simulink model "non_recursive"  (Simulink 9.1)
settings: Solver=VariableStepDiscrete  StartTime=0.0  StopTime=20.0  RelTol=1e-3  EnableMultiTasking=on
settings Model: Creator=Admin  LastModifiedBy=Asus
settings DataIOCC: LimitDataPoints=on  SignalLoggingSaveFormat=ModelDataLogs
settings OptimizationCC: ExpressionDepthLimit=2147483647  InitFltsAndDblsToZero=on
settings DebuggingCC: SaveWithParameterizedLinksMsg=none  SignalResolutionControl=TryResolveAllWithWarning  SolverPrmCheckMsg=warning  MultiTaskDSMMsg=warning  MultiTaskCondExecSysMsg=none  FcnCallInpInsideContextMsg=warning  StateNameClashWarn=warning
settings GRTTargetCC: TargetFcnLib=ansi_tfl_tmw.mat  GeneratePreprocessorConditionals=Disable all

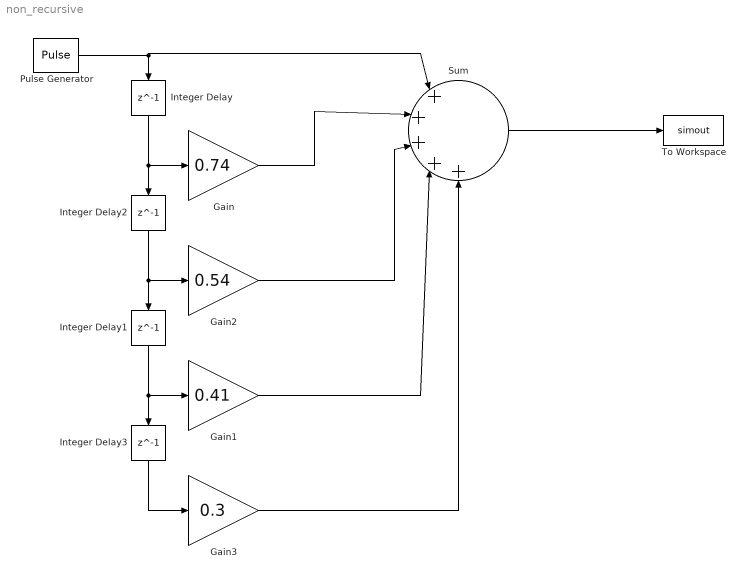
== system non_recursive ==
  Gain : Gain  Gain=0.74
  Gain1 : Gain  Gain=0.41
  Gain2 : Gain  Gain=0.54
  Gain3 : Gain  Gain=0.3
  Integer Delay{,1..3} (4 alike) : Delay  DelayLength=1  InputProcessing=Inherited
  Pulse Generator : DiscretePulseGenerator  Period=100
  Sum : Sum  Inputs=|+++++
  To Workspace : ToWorkspace  VariableName=simout  SampleTime=-1
  wires:
  Gain/1 -> Sum/2
  Sum/1 -> To Workspace/1
  Pulse Generator/1 -> Sum/1, Integer Delay/1
  Integer Delay/1 -> Integer Delay2/1, Gain/1
  Gain2/1 -> Sum/3
  Integer Delay2/1 -> Integer Delay1/1, Gain2/1
  Integer Delay1/1 -> Integer Delay3/1, Gain1/1
  Integer Delay3/1 -> Gain3/1
  Gain1/1 -> Sum/4
  Gain3/1 -> Sum/5
